simulink model "Wind_Testrig"  (Simulink 7.9)
settings: Solver=ode23t  StartTime=0.0  StopTime=400  RelTol=1e-5
PostLoadFcn:
  | warning off Simulink:blocks:MatchingGotoNotFound
  | warning off Simulink:blocks:MatchingFromNotFound
  | warning off Simulink:Engine:UsingDefaultMaxStepSize
undefined symbols (not defined in the file): Actuator_Lookup, radps2rpm, sigbuilder_block
libraries: mblibv1 x5, Wind_Lib x1, Blades_Lib x1, Pitch_Controller_Lib x1, Pitch_System_Lib x1
Description:
  | Copyright 2011 MathWorks, Inc.
settings Model: Creator=smiller  LastModifiedBy=smiller
settings DebuggingCC: FcnCallInpInsideContextMsg=Use local settings  StrictBusMsg=Warning
settings SFSimCC: SimParseCustomCode=off
settings GRTTargetCC: CombineOutputUpdateFcns=off  GRTInterface=on
settings SimMechanicsCC: AnimationDelay=0  LastVizWinPosition=[420 528 560 420]  CamPosition=[-56.1901;-28.4673;10.4676;]  CamTarget=[1.18056;0.101824;-0.229298;]  CamUpVector=[0.179671;0.00751397;0.983698;]  CamHeight=4.38469  VisBackgroundColor=[0.9;0.9;0.95;]  DefaultBodyColor=[1;0;0;]
settings ConfigurationSet: Description=SimMechanics 2G

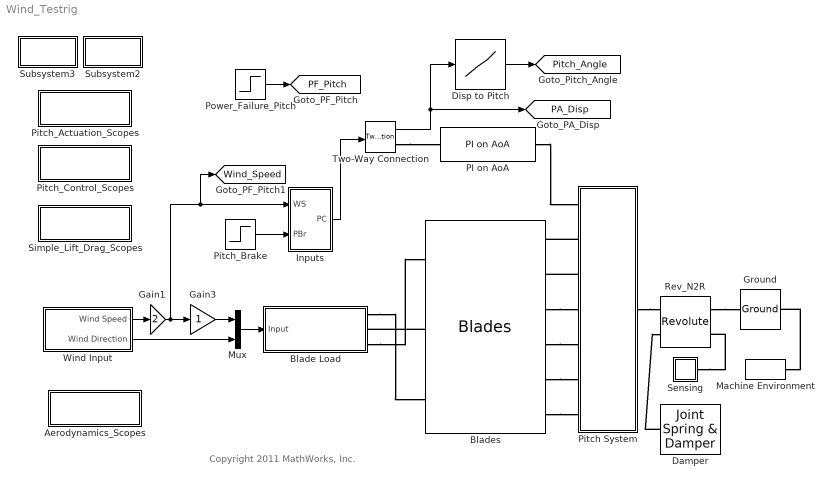
== system Wind_Testrig ==
  note: Copyright 2011 MathWorks, Inc.
  Aerodynamics_Scopes : Subsystem  AncestorBlock=Wind_Lib/Simple_Lift_Drag_Scopes
  Blade Load : Subsystem  BlockChoice=Segments
      settings: AttributesFormatString=%<BlockChoice>  TemplateBlock=Wind_Lib/Blade Load  MemberBlocks=Lift and Drag,Lift and Drag (Simscape),Segments,Torque
  Blades : Blades_Lib/Blades  SystemSampleTime=-1
  Damper : mblibv1/Force  Elements/Joint Spring & Damper  UpdateFromCAD=off  DialogClass=JointSpringDamper  JFEParameters=P1$false$0$0$0$m$m/s$N$deg$deg/s$N*m#P2$false$0$0$0$m$m/s$N$deg$deg/s$N*m#P3$false$0$0$0$m$m/s$N$deg$deg/s$N*m#R1$true$0$WT_Params.Rotor.damping$0$m$m/s$N$deg$deg/s$N*m#R2$false$0$0$0$m$m/s$N$deg$deg/s$N*m#R3$false$0$0$0$m$m/s$N$deg$deg/s$N*m#S$false$0$0$0$m$m/s$N$deg$deg/s$N*m
  Disp to Pitch : Lookup  InputValues=Actuator_Lookup.extension  Table=Actuator_Lookup.angle
  Gain1 : Gain  Gain=2
  Gain3 : Gain
  Ground : mblibv1/Bodies/Ground  UpdateFromCAD=off  LeftPortType=env  RightPortType=workingframe  PhysicalDomain=Mechanical  DialogClass=GroundBlock  CoordPosition=[0 0 0]  CoordPositionUnits=m  StateVectorMgrId=-1  MachineId=[0 0]  ShowEnvPort=on
  Inputs : Subsystem
  Machine Environment : mblibv1/Bodies/Machine Environment  PortType=env  PhysicalDomain=Mechanical  DialogTemplateClass=MECH.MachineEnvironment  SyncWhenCopied=off  Gravity=[0 -9.81 0]*0  GravityUnits=m/s^2  GravityAsSignal=off  Dimensionality=Auto-detect  AnalysisType=Forward dynamics  LinearAssemblyTolerance=1e-3  LinearAssemblyToleranceUnits=m  AngularAssemblyTolerance=1e-3  AngularAssemblyToleranceUnits=rad  ConstraintSolverType=Stabilizing  ConstraintRelTolerance=1e-4  ConstraintAbsTolerance=1e-4  UseRobustSingularityHandling=off  RedundancyAnalysisToleranceType=Specify tolerance  RedundancyAnalysisTolerance=1e-18  StatePerturbationType=Fixed  PerturbationSize=1e-5  VisualizeMachine=off  BodyVisualizationType=Use model default body geometries  BodyColorSelMode=Use model default  DefaultBodyColor=[1 0 0]
  Mux : Mux  Inputs=2
  PI on AoA : Pitch_Controller_Lib/PI on AoA  SystemSampleTime=-1
  Pitch System : Subsystem  BlockChoice=Ideal
      settings: AttributesFormatString=%<BlockChoice>  TemplateBlock=Pitch_System_Lib/Pitch System  MemberBlocks=Hydraulic,Ideal,Locked
  Pitch_Actuation_Scopes : Subsystem
  Pitch_Brake : Step  After=0  SampleTime=0
  Pitch_Control_Scopes : Subsystem
  Power_Failure_Pitch : Step  Time=5  Before=24  After=24  SampleTime=0
  Rev_N2R : mblibv1/Joints/Revolute  LConnTagsString=__newl0|SA1  RConnTagsString=__newr0|SA1  UpdateFromCAD=off  NumSAPorts=2  CutJoint=off  MarkAsCut=off  Primitives=prismatic  PrimitiveProps=R1$Base$[-1 0 0]$revolute  DialogClass=JointBlock  R1Axis=[-1 0 0]
  Sensing : Subsystem
  Simple_Lift_Drag_Scopes : Subsystem  AncestorBlock=Wind_Lib/Simple_Lift_Drag_Scopes
  Subsystem2 : Subsystem
      settings: OpenFcn=|
      | Temp_ENVHa= get_param(find_system(gcs,'LookUnderMasks','all','FollowLinks','on','ClassName','Environment'),'handle');
      | 
      | set_param(Temp_ENVHa{1},'VisualizeMachine','off');
      | 
      | set_param(gcs,'VisDuringSimulation','off')
      | set_param(gcs,'VisOnUpdateDiagram','off')
      mask Display: disp('Vis Off')
  Subsystem3 : Subsystem
      settings: OpenFcn=|
      | Temp_ENVHa= get_param(find_system(gcs,'LookUnderMasks','all','FollowLinks','on','ClassName','Environment'),'handle');
      | 
      | set_param(Temp_ENVHa{1},'VisualizeMachine','on');
      | clear Temp_ENVHa;
      | set_param(gcs,'VisDuringSimulation','on')
      | set_param(gcs,'VisOnUpdateDiagram','on')
      mask Display: disp('Vis On')
  Two-Way Connection : TwoWayConnection
  Wind Input : Subsystem  Tag=STV Subsys  LoadFcn=sigbuilder_block('load');  StartFcn=sigbuilder_block('start');  StopFcn=sigbuilder_block('stop');  ClipboardFcn=sigbuilder_block('clipboard');  mask(Sigbuilder block){}
      mask help: Sigbuilder GUI
      mask init:
      | if ~strcmp(get_param(bdroot(gcbh),'SimulationStatus'),'stopped') tuvar = sigbuilder_block('maskInit'); end
      settings: CopyFcn=sigbuilder_block('copy');  DeleteFcn=sigbuilder_block('delete');  ModelCloseFcn=sigbuilder_block('modelClose');  PreSaveFcn=sigbuilder_block('preSave');  PauseFcn=sigbuilder_block('pause')  ContinueFcn=sigbuilder_block('continue')  NameChangeFcn=sigbuilder_block('namechange');  OpenFcn=sigbuilder_block('open',[33 180 762 399.75 ]);  CloseFcn=sigbuilder_block('close');
      mask Display: plot(0,0,100,100,[10,10,40,40,10],[80,20,20,80,80],[40,10],[50,50], [40,27,10],[65,72,56],[40,25,25,10],[28,28,43,43]);
  tag scope: PA_Disp=global, PF_Pitch=global, Pitch_Angle=global, Wind_Speed=global
  wires:
  Disp to Pitch/1 -> [Pitch_Angle]
  Two-Way Connection/1 -> [PA_Disp], Disp to Pitch/1
  Power_Failure_Pitch/1 -> [PF_Pitch]
  Wind Input/1(Wind Speed) -> Gain1/1
  Wind Input/2(Wind Direction) -> Mux/2
  Mux/1 -> Blade Load/1(Input)
  Pitch_Brake/1 -> Inputs/2(PBr)
  Inputs/1(PC) -> Two-Way Connection/1
  Gain3/1 -> Mux/1
  Gain1/1 -> Gain3/1, Inputs/1(WS), [Wind_Speed]
  connections:
  Machine Environment/RConn1 -- Ground/LConn1
  Rev_N2R/RConn1 -- Ground/RConn1
  Pitch System/RConn1 -- Rev_N2R/LConn1
  Pitch System/LConn2 -- Blades/LConn1
  Blades/LConn5 -- Pitch System/LConn6
  Blades/LConn3 -- Pitch System/LConn4
  Pitch System/LConn3 -- Blades/LConn2
  Two-Way Connection/RConn1 -- PI on AoA/LConn1
  PI on AoA/RConn1 -- Pitch System/LConn1
  Blades/LConn4 -- Pitch System/LConn5
  Blades/LConn6 -- Pitch System/LConn7
  Sensing/LConn1 -- Rev_N2R/RConn2
  Damper/LConn1 -- Rev_N2R/LConn2
  Blade Load/RConn1 -- Blades/RConn3
  Blades/RConn2 -- Blade Load/RConn2
  Blade Load/RConn3 -- Blades/RConn1

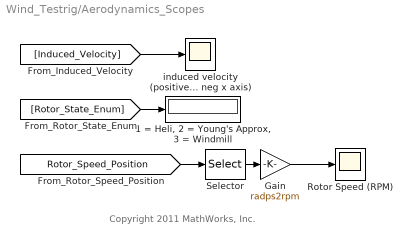
== system Wind_Testrig/Aerodynamics_Scopes ==
  note: Copyright 2011 MathWorks, Inc.
  "1 = Heli, 2 = Young's Approx, 3 = Windmill" : Display
  Gain : Gain  Gain=radps2rpm
  Rotor Speed (RPM) : Scope
      settings: TimeRange=80  YMin=0  YMax=12  SaveName=ScopeData11
  Selector : Selector  InputPortWidth=2  IndexOptions=Index vector (dialog)  Indices=[2]  OutputSizes=1
  induced velocity (positive in neg x axis) : Scope
      settings: TimeRange=100  YMin=-8  YMax=4  SaveName=ScopeData12
  wires:
  [Rotor_State_Enum] -> "1 = Heli, 2 = Young's Approx, 3 = Windmill"/1
  [Induced_Velocity] -> induced velocity (positive in neg x axis)/1
  [Rotor_Speed_Position] -> Selector/1
  Selector/1 -> Gain/1
  Gain/1 -> Rotor Speed (RPM)/1

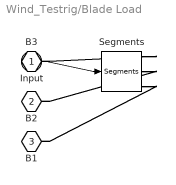
== system Wind_Testrig/Blade Load ==
  Input : Inport
  Segments : Wind_Lib/Segments  SystemSampleTime=-1
  B3 : PMIOPort  Port=1  Side=Right
  B2 : PMIOPort  Port=2  Side=Right
  B1 : PMIOPort  Port=3  Side=Right
  wires:
  Input/1 -> Segments/1
  connections:
  Segments/RConn1 -- B3/RConn1
  Segments/RConn2 -- B2/RConn1
  Segments/RConn3 -- B1/RConn1

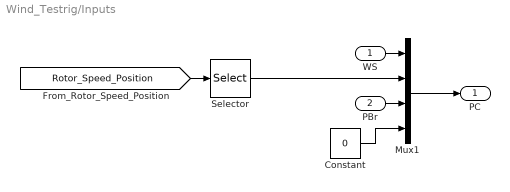
== system Wind_Testrig/Inputs ==
  WS : Inport
  PBr : Inport  Port=2
  Constant : Constant  Value=0
  Mux1 : Mux
  Selector : Selector  InputPortWidth=2  IndexOptions=Index vector (dialog)  Indices=[2]  OutputSizes=1
  PC : Outport
  wires:
  [Rotor_Speed_Position] -> Selector/1
  Selector/1 -> Mux1/2
  WS/1 -> Mux1/1
  Mux1/1 -> PC/1
  PBr/1 -> Mux1/3
  Constant/1 -> Mux1/4

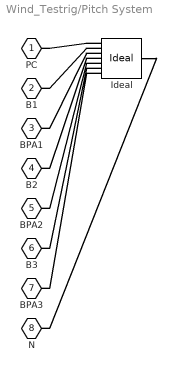
== system Wind_Testrig/Pitch System ==
  Ideal : Pitch_System_Lib/Ideal  SystemSampleTime=-1
  PC : PMIOPort  Port=1  Side=Left
  B1 : PMIOPort  Port=2  Side=Left
  BPA1 : PMIOPort  Port=3  Side=Left
  B2 : PMIOPort  Port=4  Side=Left
  BPA2 : PMIOPort  Port=5  Side=Left
  B3 : PMIOPort  Port=6  Side=Left
  BPA3 : PMIOPort  Port=7  Side=Left
  N : PMIOPort  Port=8  Side=Right
  connections:
  Ideal/LConn1 -- PC/RConn1
  Ideal/LConn2 -- B1/RConn1
  Ideal/LConn3 -- BPA1/RConn1
  Ideal/LConn4 -- B2/RConn1
  Ideal/LConn5 -- BPA2/RConn1
  Ideal/LConn6 -- B3/RConn1
  Ideal/LConn7 -- BPA3/RConn1
  Ideal/RConn1 -- N/RConn1

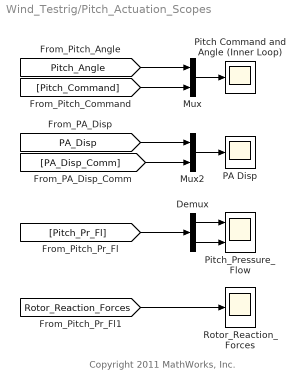
== system Wind_Testrig/Pitch_Actuation_Scopes ==
  note: Copyright 2011 MathWorks, Inc.
  Demux : Demux  Outputs=[2 1]
  Mux : Mux  Inputs=2
  Mux2 : Mux  Inputs=2
  PA Disp : Scope
      settings: TimeRange=10  YMin=-1.6  YMax=-0.9
  Pitch Command and Angle (Inner Loop) : Scope
      settings: TimeRange=400  YMin=-20  YMax=80
  Pitch_Pressure_Flow : Scope  NumInputPorts=2
      settings: TimeRange=10  YMin=-5000000~-0.005  YMax=25000000~0.015  SaveName=ScopeData3
  Rotor_Reaction_Forces : Scope
      settings: TimeRange=10  YMin=-5e+006  YMax=2.5e+007  SaveName=ScopeData15
  wires:
  [Pitch_Angle] -> Mux/1
  [Pitch_Command] -> Mux/2
  Mux/1 -> Pitch Command and Angle (Inner Loop)/1
  [PA_Disp] -> Mux2/1
  Mux2/1 -> PA Disp/1
  [PA_Disp_Comm] -> Mux2/2
  [Pitch_Pr_Fl] -> Demux/1
  Demux/1 -> Pitch_Pressure_Flow/1
  Demux/2 -> Pitch_Pressure_Flow/2
  [Rotor_Reaction_Forces] -> Rotor_Reaction_Forces/1

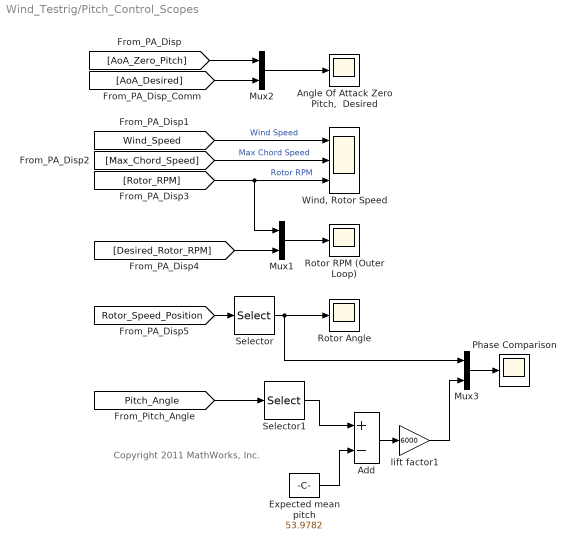
== system Wind_Testrig/Pitch_Control_Scopes ==
  note: Copyright 2011 MathWorks, Inc.
  Add : Sum  Inputs=+-
  "Angle Of Attack Zero Pitch,  Desired" : Scope
      settings: TimeRange=400  YMin=-40  YMax=100
  Expected mean pitch : Constant  Value=53.9782
  Mux1 : Mux  Inputs=2
  Mux2 : Mux  Inputs=2
  Mux3 : Mux  Inputs=2
  Phase Comparison : Scope
      settings: TimeRange=10.02528256989888  YMin=-4  YMax=4  SaveName=ScopeData16
  Rotor Angle : Scope
      settings: TimeRange=10.02528256989888  YMin=-4  YMax=4  SaveName=ScopeData7
  Rotor RPM (Outer Loop) : Scope
      settings: TimeRange=400  YMax=20  SaveName=ScopeData13
  Selector : Selector  InputPortWidth=2  IndexOptions=Index vector (dialog)  Indices=[1]  OutputSizes=1
  Selector1 : Selector  InputPortWidth=3  IndexOptions=Index vector (dialog)  Indices=[1]  OutputSizes=1
  "Wind, Rotor Speed" : Scope  NumInputPorts=3
      settings: TimeRange=600  YMin=5~-10~-10  YMax=15~20~20  SaveName=ScopeData2
  lift factor1 : Gain  Gain=6000
  wires:
  [AoA_Desired] -> Mux2/2
  Mux2/1 -> "Angle Of Attack Zero Pitch,  Desired"/1
  [AoA_Zero_Pitch] -> Mux2/1
  [Wind_Speed] -> "Wind, Rotor Speed"/1  "Wind Speed"
  [Max_Chord_Speed] -> "Wind, Rotor Speed"/2  "Max Chord Speed"
  [Rotor_RPM] -> "Wind, Rotor Speed"/3, Mux1/1  "Rotor RPM"
  Mux1/1 -> Rotor RPM (Outer Loop)/1
  [Desired_Rotor_RPM] -> Mux1/2
  [Rotor_Speed_Position] -> Selector/1
  Selector/1 -> Rotor Angle/1, Mux3/1
  Mux3/1 -> Phase Comparison/1
  Expected mean pitch/1 -> Add/2
  [Pitch_Angle] -> Selector1/1
  Selector1/1 -> Add/1
  Add/1 -> lift factor1/1
  lift factor1/1 -> Mux3/2

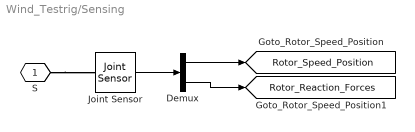
== system Wind_Testrig/Sensing ==
  Demux : Demux  Outputs=[2 3]
  Joint Sensor : mblibv1/Sensors &  Actuators/Joint Sensor  UpdateFromCAD=off  PhysicalDomain=Mechanical  PortType=blob  Muxed=on  Pose=off  Angle=on  AngleUnits=rad  ArcVelocity=on  ArcVelocityUnits=rad/s  ArcAcceleration=off  ArcAccelerationUnits=deg/s^2  CoordPosition=on  CoordPositionUnits=m  Velocity=off  VelocityUnits=m/s  Acceleration=off  AccelerationUnits=m/s^2  Quaternion=on  QuaternionDT=off  QuaternionDDT=off  QuaternionUnits=off  OutputVector=[1]  ActiveIO=on  Width=5  DialogClass=MechanicalSensorBlock  Primitive=R1  Force=off  ForceUnits=N  Torque=off  TorqueUnits=N*m  ReferenceFrame=Absolute (World)  ReactionSensedSide=Base  ReactionReferenceFrame=Absolute (World)  ReactionForce=on  ReactionForceUnits=N  ReactionMoment=off  ReactionMomentUnits=N*m
  S : PMIOPort  Tag=PMCPort  Port=1  Side=Left
  tag scope: Rotor_Reaction_Forces=global, Rotor_Speed_Position=global
  wires:
  Joint Sensor/1 -> Demux/1
  Demux/1 -> [Rotor_Speed_Position]
  Demux/2 -> [Rotor_Reaction_Forces]
  connections:
  S/RConn1 -- Joint Sensor/LConn1

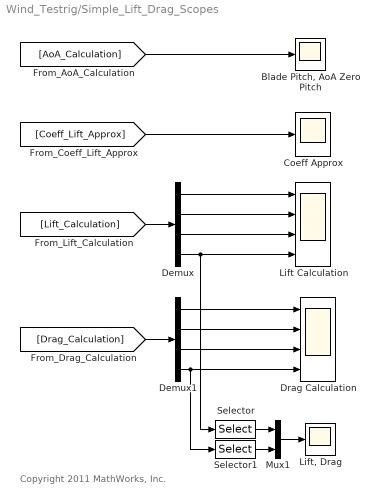
== system Wind_Testrig/Simple_Lift_Drag_Scopes ==
  note: Copyright 2011 MathWorks, Inc.
  "Blade Pitch, AoA Zero Pitch" : Scope
      settings: TimeRange=400  YMin=0  YMax=100  SaveName=ScopeData3
  Coeff Approx : Scope
      settings: TimeRange=400  YMin=-0.1139986551164904  YMax=0.01794057021302797  SaveName=ScopeData4
  Demux : Demux  Outputs=[1 3 3 3]
  Demux1 : Demux  Outputs=[1 3 3 3]
  Drag Calculation : Scope  NumInputPorts=4
      settings: TimeRange=400  YMin=-2000~-50~0~0  YMax=4000~100~6000~6000  SaveName=ScopeData5
  Lift Calculation : Scope  NumInputPorts=4
      settings: TimeRange=400  YMin=0~-50~-0.5~-50000  YMax=2000~100~1.5~100000  SaveName=ScopeData2
  "Lift, Drag" : Scope
      settings: TimeRange=160  YMin=-250.4351759669439  YMax=408.3026221352307
  Mux1 : Mux  Inputs=2
  Selector : Selector  InputPortWidth=3  IndexOptions=Index vector (dialog)  Indices=[1]  OutputSizes=1
  Selector1 : Selector  InputPortWidth=3  IndexOptions=Index vector (dialog)  Indices=[1 3]  OutputSizes=1
  wires:
  Demux1/4 -> Drag Calculation/4, Selector1/1
  Demux1/3 -> Drag Calculation/3
  Demux1/2 -> Drag Calculation/2
  Demux1/1 -> Drag Calculation/1
  [Drag_Calculation] -> Demux1/1
  [Coeff_Lift_Approx] -> Coeff Approx/1
  Demux/4 -> Lift Calculation/4, Selector/1
  Demux/3 -> Lift Calculation/3
  Demux/2 -> Lift Calculation/2
  Demux/1 -> Lift Calculation/1
  [Lift_Calculation] -> Demux/1
  Mux1/1 -> "Lift, Drag"/1
  [AoA_Calculation] -> "Blade Pitch, AoA Zero Pitch"/1
  Selector/1 -> Mux1/1
  Selector1/1 -> Mux1/2

== system Wind_Testrig/Subsystem2 ==

== system Wind_Testrig/Subsystem3 ==

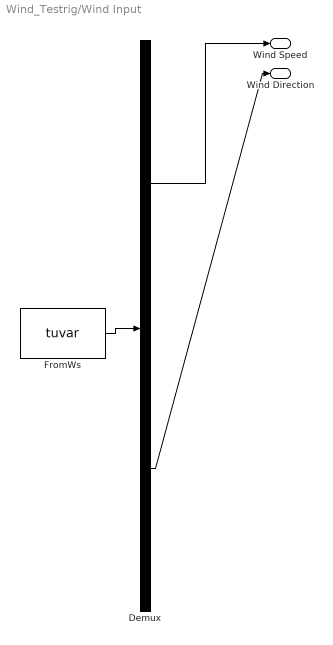
== system Wind_Testrig/Wind Input ==
  Demux : Demux  Tag=STV Demux  Outputs=2
  FromWs : FromWorkspace  Tag=STV FromWs  VariableName=tuvar  SampleTime=0  SigBuilderData=DataTag1  VnvData=DataTag2
      SigBuilderData=|
      | common.afterFinalStr = 'Extrapolate'
      | common.sampleTime = 0
      | dataSet(1).timeRange = [0 130]
      | dataSet(1).name = 'High Wind Speed'
      | dataSet(2).timeRange = [0 130]
      | dataSet(2).name = 'Constant Wind'
      | dataSet(3).timeRange = [0 130]
      | dataSet(3).name = 'Cut In'
      | sbobj.Groups(1).Name = 'High Wind Speed'
      | sbobj.Groups(1).Signals(1).Name = 'Wind Speed'
      | sbobj.Groups(1).Signals(1).XData = [0 10 10 25.1 28 91.8 100 130]
      | sbobj.Groups(1).Signals(1).YData = [10 10 9.9 9.9 5 5 8 10]
      | sbobj.Groups(1).Signals(2).Name = 'Wind Direction'
      | sbobj.Groups(1).Signals(2).XData = [0 1 1 11 11 21 21 31 31 130]
      | sbobj.Groups(1).Signals(2).YData = [0 0 4 4 0 0 -4 -4 0 0]
      | sbobj.Groups(2).Name = 'Constant Wind'
      | sbobj.Groups(2).Signals(1).Name = 'Wind Speed'
      | sbobj.Groups(2).Signals(1).XData = [0 10 130]
      | sbobj.Groups(2).Signals(1).YData = [10 10 10]
      | sbobj.Groups(2).Signals(2).Name = 'Wind Direction'
      | sbobj.Groups(2).Signals(2).XData = [0 1 1 11 11 21 21 31 31 130]
      | sbobj.Groups(2).Signals(2).YData = [0 0 4 4 0 0 -4 -4 0 0]
      | sbobj.Groups(3).Name = 'Cut In'
      | sbobj.Groups(3).Signals(1).Name = 'Wind Speed'
      | sbobj.Groups(3).Signals(1).XData = [0 25.1 28 91.8 100 121.8 130]
      | sbobj.Groups(3).Signals(1).YData = [4.5 8.7 7.85 9.65 8 10 10]
      | sbobj.Groups(3).Signals(2).Name = 'Wind Direction'
      | sbobj.Groups(3).Signals(2).XData = [0 1 1 11 11 21 21 31 31 130]
      | sbobj.Groups(3).Signals(2).YData = [0 0 4 4 0 0 -4 -4 0 0]
  Wind Speed : Outport  Tag=STV Outport
  Wind Direction : Outport  Tag=STV Outport  Port=2
  wires:
  Demux/2 -> Wind Direction/1
  Demux/1 -> Wind Speed/1
  FromWs/1 -> Demux/1
